simulink model "lab3vase"  (R2013b)
settings: Solver=ode45  StartTime=0.0  StopTime=10.0  RelTol=1e-3
settings Model: Creator=User  LastModifiedBy=User

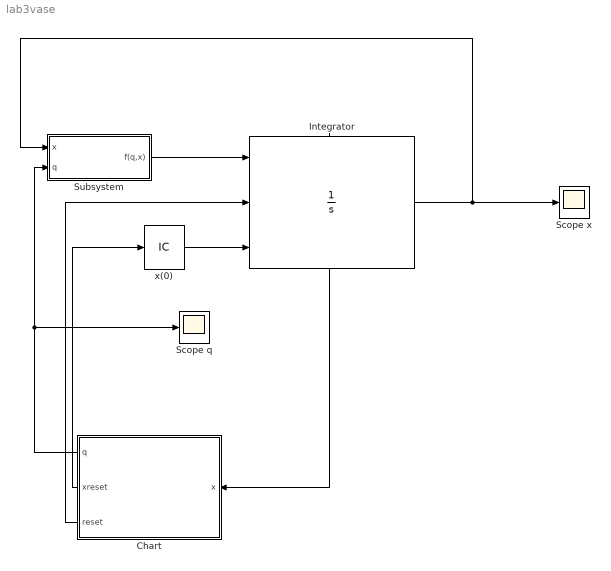
== system lab3vase ==
  Chart : Stateflow chart  TreatAsAtomicUnit=on
  Integrator : Integrator  ExternalReset=rising  InitialConditionSource=external  LimitOutput=on  LowerSaturationLimit=[0;-inf]  ShowStatePort=on
  Scope q : Scope
  Scope x : Scope
  Subsystem : Subsystem
  x(0) : InitialCondition  Value=[10;10]
  wires:
  Integrator/State -> Chart/1(x)
  Subsystem/1(f(q,x)) -> Integrator/1
  x(0)/1 -> Integrator/3
  Chart/3(reset) -> Integrator/2
  Chart/2(xreset) -> x(0)/1
  Chart/1(q) -> Scope q/1, Subsystem/2(q)
  Integrator/1 -> Subsystem/1(x), Scope x/1

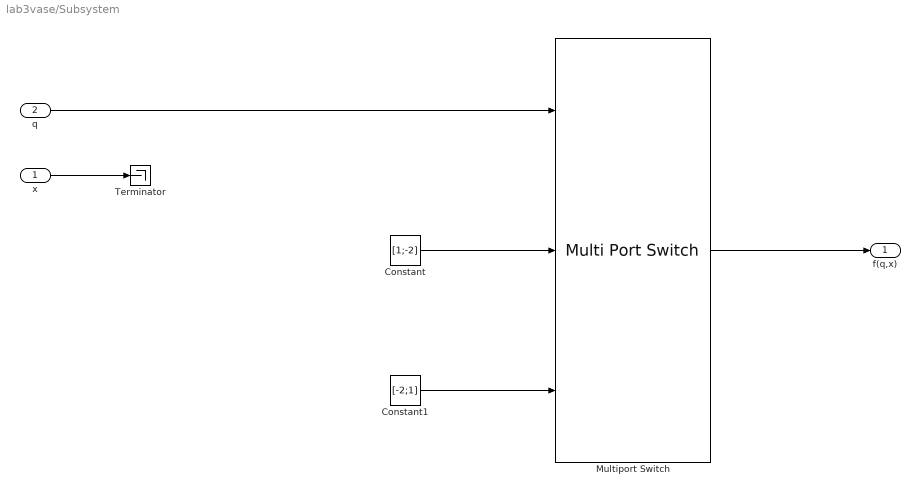
== system lab3vase/Subsystem ==
  x : Inport
  q : Inport  Port=2
  Constant : Constant  Value=[1;-2]
  Constant1 : Constant  Value=[-2;1]
  Multiport Switch : MultiPortSwitch  Inputs=2
  Terminator : Terminator
  f(q,x) : Outport
  wires:
  q/1 -> Multiport Switch/1
  Multiport Switch/1 -> f(q,x)/1
  x/1 -> Terminator/1
  Constant/1 -> Multiport Switch/2
  Constant1/1 -> Multiport Switch/3

== stateflow chart lab3vase/Chart ==
  state tank1/
    entry:q=1;
  state tank2/
    entry:q=2;
  (default) -> tank1
  tank2 -> tank1 : [x[1]<=5]/
      | xreset[1]=x[1];
      | xreset[2]=x[2];
      | reset
  tank1 -> tank2 : [x[2]<=5]/
      | xreset[1]=x[1];
      | xreset[2]=x[2];
      | reset
  data: x input double size=2; q output double; xreset output double size=2
  data x settings: description=1
  data xreset settings: description=1
  events: reset output EITHER_EDGE_EVENT
